simulink model "SD_Card_SPI_Demo"  (R2024b)
settings: Solver=FixedStepAuto  StartTime=0.0  StopTime=2.0  FixedStep=0.1  RelTol=1e-3
settings Model: Creator=Shreyas  LastModifiedBy=Shreyas
settings SFSimCC: SimCustomSourceCode="#include \"sd_spi.c\""  SimCustomHeaderCode="#include \"sd_spi.h\""
settings RTWCC: CustomSourceCode="#include \"sd_spi.c\""  CustomHeaderCode="#include \"sd_spi.h\""

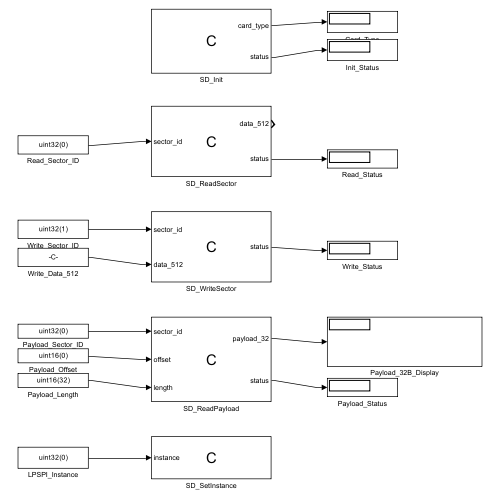
[thumbnail: Simulink's stored preview of the top-level diagram]
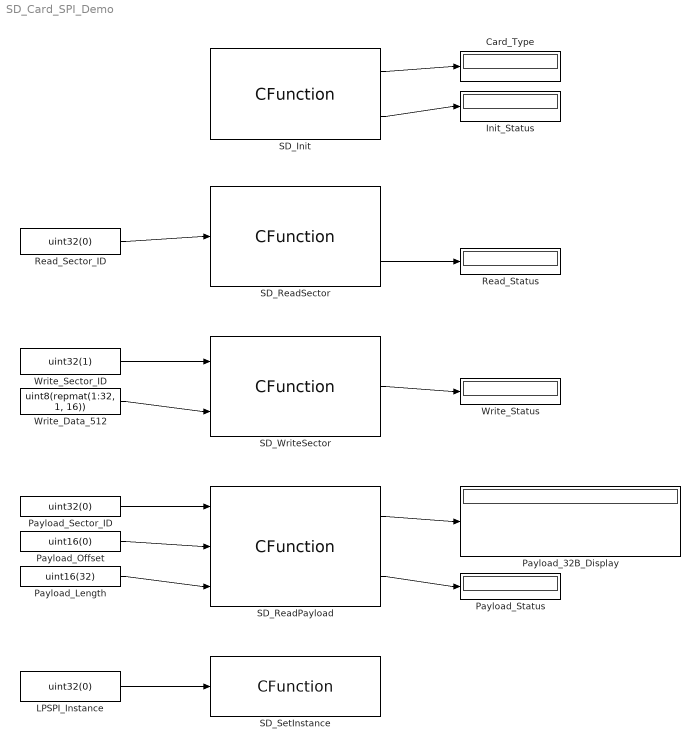
== system SD_Card_SPI_Demo ==
  Card_Type : Display
  Init_Status : Display
  LPSPI_Instance : Constant  Value=uint32(0)  OutDataTypeStr=uint32
  Payload_32B_Display : Display
  Payload_Length : Constant  Value=uint16(32)  OutDataTypeStr=uint16
  Payload_Offset : Constant  Value=uint16(0)  OutDataTypeStr=uint16
  Payload_Sector_ID : Constant  Value=uint32(0)  OutDataTypeStr=uint32
  Payload_Status : Display
  Read_Sector_ID : Constant  Value=uint32(0)  OutDataTypeStr=uint32
  Read_Status : Display
  SD_Init : CFunction  OutputCode=|  CodegenOutputCode=|  SimCustomHeaderFile=sd_spi.h  SimCustomSourceFile=sd_spi.c  CustomHeaderFile=sd_spi.h  CustomSourceFile=sd_spi.c  CustomCodeIsMultiInstantiable=on
      OutputCode=|
      | /* Initialize SD Card over SPI */
      | status = SD_Init();
      | card_type = SD_GetCardType();
      CodegenOutputCode=|
      | /* Initialize SD Card over SPI */
      | status = SD_Init();
      | card_type = SD_GetCardType();
  SD_ReadPayload : CFunction  OutputCode=|  CodegenOutputCode=|  SimCustomHeaderFile=sd_spi.h  SimCustomSourceFile=sd_spi.c  CustomHeaderFile=sd_spi.h  CustomSourceFile=sd_spi.c  CustomCodeIsMultiInstantiable=on
      OutputCode=|
      | /* Read Partial Payload from Sector (e.g. 32-Byte BMS Record) */
      | status = SD_ReadPayload(sector_id, offset, payload_32, length);
      CodegenOutputCode=|
      | /* Read Partial Payload from Sector (e.g. 32-Byte BMS Record) */
      | status = SD_ReadPayload(sector_id, offset, payload_32, length);
  SD_ReadSector : CFunction  OutputCode=|  CodegenOutputCode=|  SimCustomHeaderFile=sd_spi.h  SimCustomSourceFile=sd_spi.c  CustomHeaderFile=sd_spi.h  CustomSourceFile=sd_spi.c  CustomCodeIsMultiInstantiable=on
      OutputCode=|
      | /* Read Single 512-Byte Physical Sector */
      | status = SD_ReadSector(sector_id, data_512);
      CodegenOutputCode=|
      | /* Read Single 512-Byte Physical Sector */
      | status = SD_ReadSector(sector_id, data_512);
  SD_SetInstance : CFunction  OutputCode=|  CodegenOutputCode=|  SimCustomHeaderFile=sd_spi.h  SimCustomSourceFile=sd_spi.c  CustomHeaderFile=sd_spi.h  CustomSourceFile=sd_spi.c  CustomCodeIsMultiInstantiable=on
      OutputCode=|
      | /* Configure LPSPI Instance (0 = LPSPI0, 1 = LPSPI1, 2 = LPSPI2) */
      | SD_SetSPIInstance(instance);
      CodegenOutputCode=|
      | /* Configure LPSPI Instance (0 = LPSPI0, 1 = LPSPI1, 2 = LPSPI2) */
      | SD_SetSPIInstance(instance);
  SD_WriteSector : CFunction  OutputCode=|  CodegenOutputCode=|  SimCustomHeaderFile=sd_spi.h  SimCustomSourceFile=sd_spi.c  CustomHeaderFile=sd_spi.h  CustomSourceFile=sd_spi.c  CustomCodeIsMultiInstantiable=on
      OutputCode=|
      | /* Write Single 512-Byte Physical Sector */
      | status = SD_WriteSector(sector_id, data_512);
      CodegenOutputCode=|
      | /* Write Single 512-Byte Physical Sector */
      | status = SD_WriteSector(sector_id, data_512);
  Write_Data_512 : Constant  Value=uint8(repmat(1:32, 1, 16))  OutDataTypeStr=uint8
  Write_Sector_ID : Constant  Value=uint32(1)  OutDataTypeStr=uint32
  Write_Status : Display
  wires:
  SD_Init/1 -> Card_Type/1
  SD_Init/2 -> Init_Status/1
  Read_Sector_ID/1 -> SD_ReadSector/1
  SD_ReadSector/2 -> Read_Status/1
  Write_Sector_ID/1 -> SD_WriteSector/1
  Write_Data_512/1 -> SD_WriteSector/2
  SD_WriteSector/1 -> Write_Status/1
  Payload_Sector_ID/1 -> SD_ReadPayload/1
  Payload_Offset/1 -> SD_ReadPayload/2
  Payload_Length/1 -> SD_ReadPayload/3
  SD_ReadPayload/1 -> Payload_32B_Display/1
  SD_ReadPayload/2 -> Payload_Status/1
  LPSPI_Instance/1 -> SD_SetInstance/1
